simulink model "TemperatureInAroom"  (R2019a)
settings: Solver=VariableStepAuto  StartTime=0.0  StopTime=T  MaxStep=MaxStep  RelTol=RelTol
values from neighbouring files (symbols this model uses):
  T = 10    [init.m]
  x0 = 55    [init.m]
undefined symbols (not defined in the file or in its folder): sigbuilder_block
libraries: HyEQ_Library x1
settings Model: Creator=HAASTRUP ADEBAYO  LastModifiedBy=HAASTRUP ADEBAYO

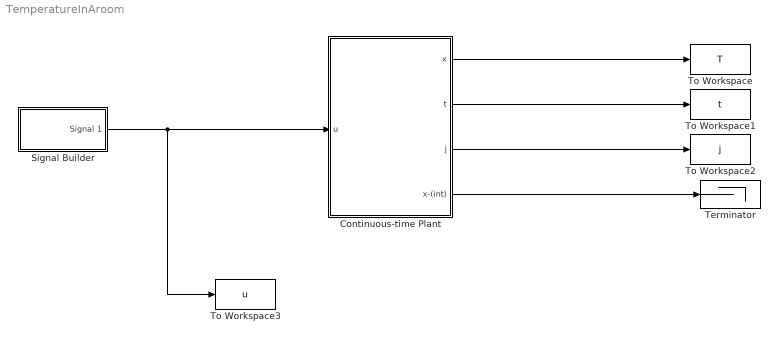
== system TemperatureInAroom ==
  Continuous-time Plant : Subsystem  LoadFcn=set_param(gcb,'LinkStatus','none')  mask(Continuous Process){z0=x0, input_dim=1, parameters=[], T=T}
      mask prompts: z0 "Initial State (column vector)"; input_dim "Input dimension (nonnegative integer)"; T "Flow Horizon (nonnegative real)"
      mask help:
      | To define the continuous process:
      | 1. Select the block,
      | 2. "Look inside" the block: Either open the context menu and select Mask > Look Under Mask, or click the arrow in the bottom-left corner of the block.
      | 3. Edit the "flow map f" block to define the continuous dynamics.
      | 4. Edit the "flow set C" block to define the region where the continuous process is allowed to flow.
      mask init:
      | state_dim = size(z0, 1);
      settings: CopyFcn=|
      | set_param(gcb,'LinkStatus','none'),
      | set_param(gcs, 'MaxStep', 'MaxStep', 'RelTol', 'RelTol','StopTime', 'T')
      mask Help: eval hybrid.internal.openHelp('Example_vehicle_on_path')
      mask TypeOptions T: Integrator System/T
      mask DialogControl Control2 Prompt: CPS Components Documentation
      mask DialogControl Control2 Callback: hybrid.internal.openHelp('CPS_Components')
      mask DialogControl ParameterGroupVar Prompt: Configuration
      mask Display:
      | image('Cplant.jpg')
      | port_label('output', 1, 'x')
      | port_label('output', 2, 't')
      | port_label('output', 3, 'j')
      | port_label('output', 4, 'x-(int)')
      | port_label('input', 1, 'u')
  Signal Builder : Subsystem  Tag=STV Subsys  LoadFcn=sigbuilder_block('load');  StartFcn=sigbuilder_block('start');  StopFcn=sigbuilder_block('stop');  ClipboardFcn=sigbuilder_block('clipboard');  mask(Sigbuilder block){tuvar=[0:10]}
      mask help: Simulink:masks:SigbuilderBlock_MD
      mask init:
      | if ~strcmp(get_param(bdroot(gcbh),'SimulationStatus'),'stopped') tuvar = sigbuilder_block('maskInit'); end
      settings: CopyFcn=sigbuilder_block('copy');  DeleteFcn=sigbuilder_block('delete');  ModelCloseFcn=sigbuilder_block('modelClose');  PreSaveFcn=sigbuilder_block('preSave');  PauseFcn=sigbuilder_block('pause');  ContinueFcn=sigbuilder_block('continue');  NameChangeFcn=sigbuilder_block('namechange');  OpenFcn=sigbuilder_block('open',[437.6 199.2 550.4 400 ]);  CloseFcn=sigbuilder_block('close');
      mask Display: plot(0, 0, 100, 100,[2, 2, 32, 32, 2], [68, 8, 8, 68, 68],[32, 2], [38, 38], [32, 19, 2],[53, 60, 44], [32, 17, 17, 2],[16, 16, 31, 31]);txt = getActiveGroup(gcbh);text(2, 100, txt,'verticalAlignment', 'top');
  Terminator : Terminator
  To Workspace : ToWorkspace  VariableName=T  SampleTime=-1
  To Workspace1 : ToWorkspace  VariableName=t  SampleTime=-1
  To Workspace2 : ToWorkspace  VariableName=j  SampleTime=-1
  To Workspace3 : ToWorkspace  VariableName=u  SampleTime=-1
  wires:
  Continuous-time Plant/1(x) -> To Workspace/1
  Continuous-time Plant/2(t) -> To Workspace1/1
  Continuous-time Plant/3(j) -> To Workspace2/1
  Continuous-time Plant/4(x-(int)) -> Terminator/1
  Signal Builder/1(Signal 1) -> To Workspace3/1, Continuous-time Plant/1(u)

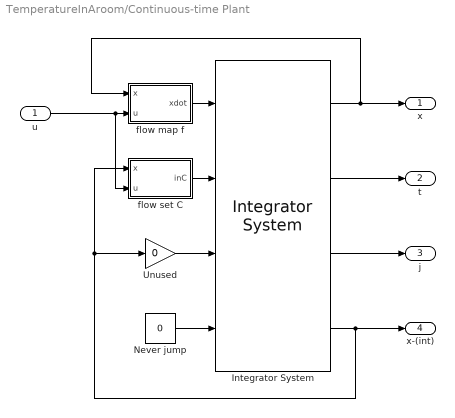
== system TemperatureInAroom/Continuous-time Plant ==
  u : Inport  PortDimensions=input_dim
  Integrator System : HyEQ_Library/Other/Integrator System  Priority=2  T=T  J=1  x0=z0  rule=1
      settings: SourceProductName=Hybrid Equations Toolbox
  Never jump : Constant  Value=0
  Unused : Gain  Gain=0
  flow map f : MATLAB Function  TreatAsAtomicUnit=on
  flow set C : MATLAB Function  TreatAsAtomicUnit=on
  x : Outport  PortDimensions=state_dim
  t : Outport  Port=2  PortDimensions=1
  j : Outport  Port=3  PortDimensions=1
  x-(int) : Outport  Port=4  PortDimensions=state_dim
  wires:
  Unused/1 -> Integrator System/3
  Never jump/1 -> Integrator System/4
  u/1 -> flow map f/2(u), flow set C/2(u)
  Integrator System/3 -> j/1
  Integrator System/2 -> t/1
  flow set C/1(inC) -> Integrator System/2
  Integrator System/1 -> x/1, flow map f/1(x)
  Integrator System/4 -> x-(int)/1, flow set C/1(x), Unused/1
  flow map f/1(xdot) -> Integrator System/1

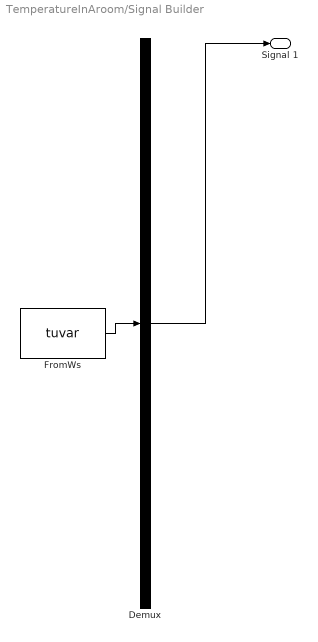
== system TemperatureInAroom/Signal Builder ==
  Demux : Demux  Tag=STV Demux  Outputs=1
  FromWs : FromWorkspace  Tag=STV FromWs  VariableName=tuvar  SampleTime=0
      SigBuilderData=|
      | common.afterFinalStr = 'Extrapolate'
      | common.sampleTime = 0
      | dataSet.timeRange = [0 10]
      | dataSet.name = 'Group 1'
      | sbobj.Groups.Name = 'Group 1'
      | sbobj.Groups.Signals.Name = 'Signal 1'
      | sbobj.Groups.Signals.XData = [0 4 4 6 6 10]
      | sbobj.Groups.Signals.YData = [0 0 1 1 0 0]
  Signal 1 : Outport  Tag=STV Outport
  wires:
  Demux/1 -> Signal 1/1
  FromWs/1 -> Demux/1

== matlab function TemperatureInAroom/Continuous-time Plant/flow map f ==
  data: x input size=state_dim; xdot output size=state_dim; u input size=input_dim
function xdot = f(x, u)
% Define the flow map for the continuous process here.
%a=parameters(1);
%Tr=parameters(2);
%Tdelta=parameters(3);
a=1;
Tr=65;
Tdelta=20;
T=x;
Tdot=-a*T+Tr+Tdelta*u;

xdot =Tdot;

== matlab function TemperatureInAroom/Continuous-time Plant/flow set C ==
  data: x input size=state_dim; inC output size=1; u input size=input_dim
function inC = C(x, u)
    % Define the flow set indicator function for the continuous process here.
    inC = 1;
end
